simulink model "Control_Model_Simulink_2"  (R2021a)
settings: Solver=VariableStepAuto  StartTime=0.0  StopTime=10.0  RelTol=1e-3
values from neighbouring files (symbols this model uses):
  A = []    [Fixed_Model.m]    (also in Matlab_Linear_Model.m = [0 1 ; 0 -Br/I]; Matlab__Linear_Model.m = [0 1 ; 0 Br/I]; Matlab__Linear_Model_2.m = [0 1 ; 0 -Br/I]; Matlab__NonLinear_Model.m = [0 1 ; 0 Br/I])
  B = []    [Fixed_Model.m]    (also in Matlab_Linear_Model.m = [0 ;1]; Matlab__Linear_Model.m = [0 0 ; 1/I -l2x/I]; Matlab__Linear_Model_2.m = [0 0 ; -F2/I 1]; Matlab__NonLinear_Model.m = [0 0 ; -H/I -l2x/I])
  C = [1 0]    [Matlab_Linear_Model.m]    (also in Matlab__Linear_Model.m; Matlab__Linear_Model_2.m; Matlab__NonLinear_Model.m; Mc1.mat)
  K = lqr(A,B,Q,R)    [Matlab_Linear_Model.m]    (also in Matlab__Linear_Model.m; Matlab__Linear_Model_2.m; Mc1.mat = [1 0.446480452821]; initialize.m)
settings Model: Creator=DANI-TUF  LastModifiedBy=DANI-TUF

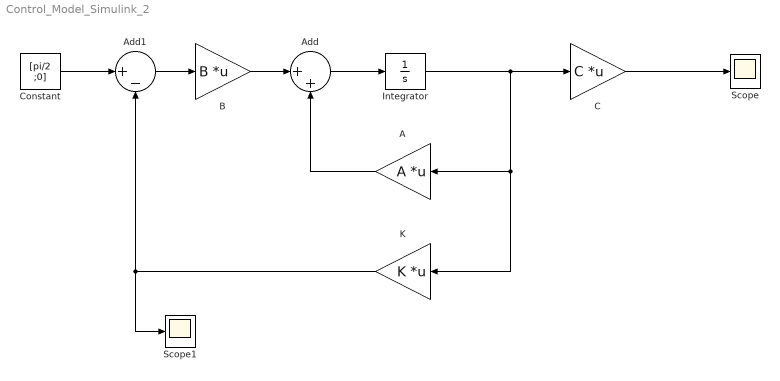
== system Control_Model_Simulink_2 ==
  A : Gain  Gain=A  Multiplication=Matrix(K*u)
  Add : Sum  Inputs=|++
  Add1 : Sum  Inputs=|+-
  B : Gain  Gain=B  Multiplication=Matrix(K*u)
  C : Gain  Gain=C  Multiplication=Matrix(K*u)
  Constant : Constant  Value=[pi/2 ;0]
  Integrator : Integrator
  K : Gain  Gain=K  Multiplication=Matrix(K*u)
  Scope : Scope
  Scope1 : Scope
  wires:
  Add/1 -> Integrator/1
  A/1 -> Add/2
  K/1 -> Scope1/1, Add1/2
  Add1/1 -> B/1
  B/1 -> Add/1
  Constant/1 -> Add1/1
  C/1 -> Scope/1
  Integrator/1 -> C/1, A/1, K/1
